simulink model "ClarkTransforms_harness"  (R2020a)
settings: Solver=VariableStepAuto  StartTime=0.0  StopTime=0.05  RelTol=1e-3
libraries: ElectricalModelLib x2, simulink x2
settings Model: Creator=cleme  LastModifiedBy=cleme

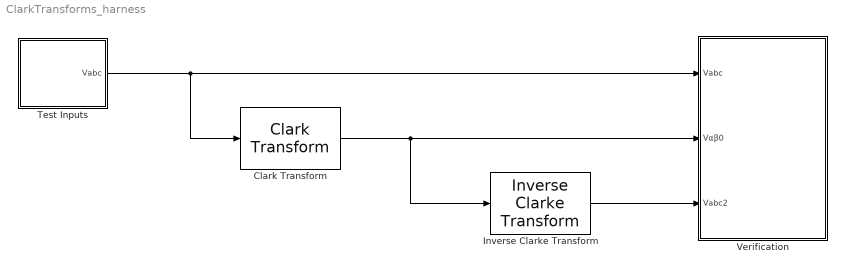
== system ClarkTransforms_harness ==
  Clark Transform : ElectricalModelLib/Clark Transform
  Inverse Clarke Transform : ElectricalModelLib/Inverse Clarke Transform
  Test Inputs : Subsystem
  Verification : Subsystem
  wires:
  Clark Transform/1 -> Inverse Clarke Transform/1, Verification/2(Vαβ0)
  Inverse Clarke Transform/1 -> Verification/3(Vabc2)
  Test Inputs/1(Vabc) -> Clark Transform/1, Verification/1(Vabc)

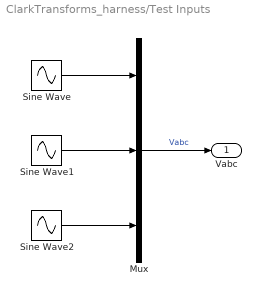
== system ClarkTransforms_harness/Test Inputs ==
  Mux : Mux  Inputs=3
  Sine Wave : Sin  Frequency=2*pi*3/0.05  SampleTime=0
  Sine Wave1 : Sin  Frequency=2*pi*3/0.05  Phase=-2*pi()/3  SampleTime=0
  Sine Wave2 : Sin  Frequency=2*pi*3/0.05  Phase=2*pi()/3  SampleTime=0
  Vabc : Outport
  wires:
  Sine Wave2/1 -> Mux/3
  Sine Wave1/1 -> Mux/2
  Sine Wave/1 -> Mux/1
  Mux/1 -> Vabc/1  "Vabc"

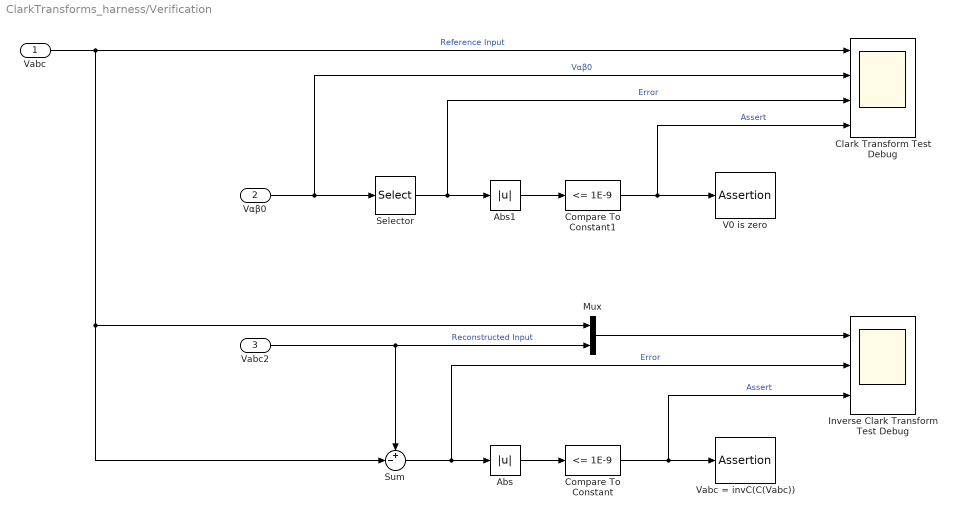
== system ClarkTransforms_harness/Verification ==
  Vabc : Inport
  Vαβ0 : Inport  Port=2
  Vabc2 : Inport  Port=3
  Abs : Abs
  Abs1 : Abs
  Clark Transform Test Debug : Scope  NumInputPorts=4
  Compare To Constant : simulink/Logic and Bit Operations/Compare To Constant  relop=<=  const=1E-9  OutDataTypeStr=boolean
  Compare To Constant1 : simulink/Logic and Bit Operations/Compare To Constant  relop=<=  const=1E-9  OutDataTypeStr=boolean
  Inverse Clark Transform Test Debug : Scope  NumInputPorts=3
  Mux : Mux  Inputs=2
  Selector : Selector  InputPortWidth=3  IndexOptions=Index vector (dialog)  Indices=3  OutputSizes=1
  Sum : Sum  Inputs=+-|
  V0 is zero : Assertion
  "Vabc = invC(C(Vabc))  " : Assertion
  wires:
  Abs/1 -> Compare To Constant/1
  Compare To Constant1/1 -> Clark Transform Test Debug/4, V0 is zero/1  "Assert"
  Vαβ0/1 -> Clark Transform Test Debug/2, Selector/1  "Vαβ0"
  Vabc/1 -> Mux/1, Sum/2, Clark Transform Test Debug/1  "Reference Input"
  Sum/1 -> Inverse Clark Transform Test Debug/2, Abs/1  "Error"
  Selector/1 -> Abs1/1, Clark Transform Test Debug/3  "Error"
  Compare To Constant/1 -> Inverse Clark Transform Test Debug/3, "Vabc = invC(C(Vabc))  "/1  "Assert"
  Vabc2/1 -> Sum/1, Mux/2  "Reconstructed Input"
  Mux/1 -> Inverse Clark Transform Test Debug/1
  Abs1/1 -> Compare To Constant1/1
